simulink model "Labaa3"  (R2017b)
settings: Solver=VariableStepAuto  StartTime=0.0  StopTime=10.0  RelTol=1e-3
undefined symbols (not defined in the file): qammod
libraries: commfilt2 x2, commchan3 x1, commrflib2 x1, dspsigops x1, dspstat3 x1, commsink2 x1, commrandsrc3 x1
settings Model: Creator=Дима  LastModifiedBy=Lab
settings DataIOCC: ReturnWorkspaceOutputs=on
settings DebuggingCC: UnconnectedInputMsg=none  UnconnectedOutputMsg=none  UnconnectedLineMsg=none
settings ModelReferenceCC: EnableRefExpFcnMdlSchedulingChecks=off
settings SFSimCC: SimUseLocalCustomCode=on
settings RTWCC: Description=Generic Real-Time Target  RTWUseLocalCustomCode=on

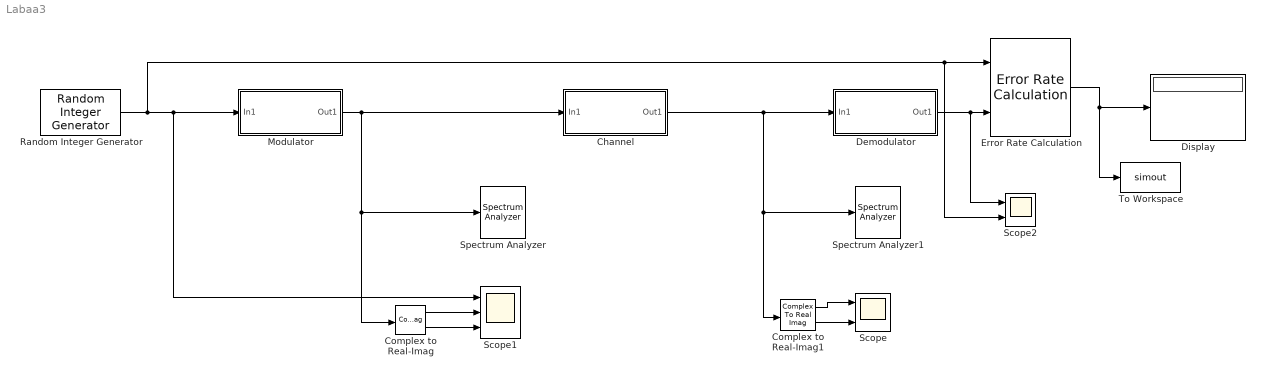
== system Labaa3 ==
  Channel : Subsystem
  Complex to Real-Imag : ComplexToRealImag
  Complex to Real-Imag1 : ComplexToRealImag
  Demodulator : Subsystem
  Display : Display
  Error Rate Calculation : commsink2/Error Rate Calculation  N=0  st_delay=0  cp_mode=Entire frame  subframe=[]  PMode=Port  WsName=ErrorVec  RsMode2=off  stop=off  numErr=100  maxBits=1e6
  Modulator : Subsystem
  Random Integer Generator : commrandsrc3/Random Integer Generator  SetSize=8  SeedSource=Auto  Seed=0  SampleTime=1/9600  SamplesPerFrame=1  OutputDataType=double  SimulateUsing=Interpreted execution
  Scope : Scope  NumInputPorts=2
  Scope1 : Scope  NumInputPorts=3
  Scope2 : Scope  NumInputPorts=2
  Spectrum Analyzer : SpectrumAnalyzer
  Spectrum Analyzer1 : SpectrumAnalyzer
  To Workspace : ToWorkspace  VariableName=simout  SaveFormat=Timeseries  SampleTime=-1
  wires:
  Complex to Real-Imag1/2 -> Scope/2
  Complex to Real-Imag1/1 -> Scope/1
  Modulator/1(Out1) -> Channel/1(In1), Complex to Real-Imag/1, Spectrum Analyzer/1
  Random Integer Generator/1 -> Scope2/2, Error Rate Calculation/1, Modulator/1(In1), Scope1/1
  Complex to Real-Imag/2 -> Scope1/3
  Complex to Real-Imag/1 -> Scope1/2
  Channel/1(Out1) -> Demodulator/1(In1), Complex to Real-Imag1/1, Spectrum Analyzer1/1
  Demodulator/1(Out1) -> Scope2/1, Error Rate Calculation/2
  Error Rate Calculation/1 -> To Workspace/1, Display/1

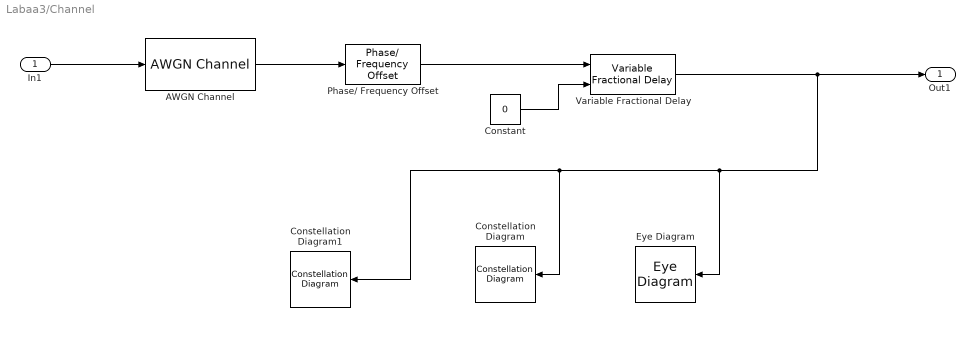
== system Labaa3/Channel ==
  In1 : Inport
  AWGN Channel : commchan3/AWGN Channel  InputProcessing=Inherited (this choice will be removed - see release notes)  seed=67  noiseMode="Signal to noise ratio  (SNR)"  EbNodB=10  EsNodB=10  SNRdB=13  bitsPerSym=1  Ps=1  Tsym=1  variance=1
  Constant : Constant  Value=0
  Constellation Diagram : ConstellationDiagram
  Constellation Diagram1 : ConstellationDiagram
  Eye Diagram : EyeDiagram
  Phase/ Frequency Offset : commrflib2/Phase// Frequency Offset  phaseOffset=0  freqPort=off  freqOffset=0
      settings: SourceProductName=Communications System Toolbox
  Variable Fractional Delay : dspsigops/Variable Fractional Delay  mode=OBSOLETE  modeActive=Linear  dmax=100  InputProcessing=Columns as channels (frame based)  L=4  FarrowL=4  R=10  alpha=1  ic=0  fallbackFIR=Clip to the minimum value necessary for centered kernel  fallbackFarrow=Clip to the minimum value necessary for centered kernel  noDFT=off  roundingMode=Zero  overflowMode=off
      settings: SourceProductName=DSP System Toolbox  SourceProductBaseCode=DS
  Out1 : Outport  VectorParamsAs1DForOutWhenUnconnected=on
  wires:
  In1/1 -> AWGN Channel/1
  AWGN Channel/1 -> Phase/ Frequency Offset/1
  Phase/ Frequency Offset/1 -> Variable Fractional Delay/1
  Constant/1 -> Variable Fractional Delay/2
  Variable Fractional Delay/1 -> Constellation Diagram/1, Constellation Diagram1/1, Eye Diagram/1, Out1/1

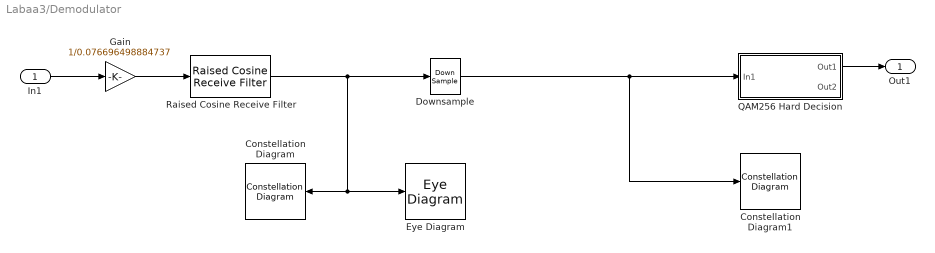
== system Labaa3/Demodulator ==
  In1 : Inport
  Constellation Diagram : ConstellationDiagram
  Constellation Diagram1 : ConstellationDiagram
  Downsample : DownSample  N=8  RateOptions=Allow multirate processing
  Eye Diagram : EyeDiagram
  Gain : Gain  Gain=1/0.076696498884737
  QAM256 Hard Decision : Subsystem
  Raised Cosine Receive Filter : commfilt2/Raised Cosine Receive Filter  filtType=Square root  R=0.8  filtSpan=10  N=8  downFactor=8  downOffset=0  filterGain=1  RateOptions=Allow multirate processing  framing=Mute  checkCoeff=off  variableName=rcRxFilt  currentFiltSpan=10  D=5  inputOffset=0  sampMode=Mute  saveAsFlag=0  rateMode=Downsampling  checkGain=Normalized  launchFVT=on  roundingMode=Floor  overflowMode=off  coeffDataTypeStr=Inherit: Same word length as input  coeffMin=[]  coeffMax=[]  coeffLastDataTypeStr=Inherit: Same word length as input  accumDataTypeStr=Inherit: Same as product output  accumLastDataTypeStr=Inherit: Same as product output  outputDataTypeStr=Inherit: Same as accumulator  outputMin=[]  outputMax=[]  outputLastDataTypeStr=Inherit: Same as accumulator
  Out1 : Outport  VectorParamsAs1DForOutWhenUnconnected=on
  wires:
  In1/1 -> Gain/1
  Gain/1 -> Raised Cosine Receive Filter/1
  Raised Cosine Receive Filter/1 -> Constellation Diagram/1, Eye Diagram/1, Downsample/1
  Downsample/1 -> Constellation Diagram1/1, QAM256 Hard Decision/1(In1)
  QAM256 Hard Decision/1(Out1) -> Out1/1

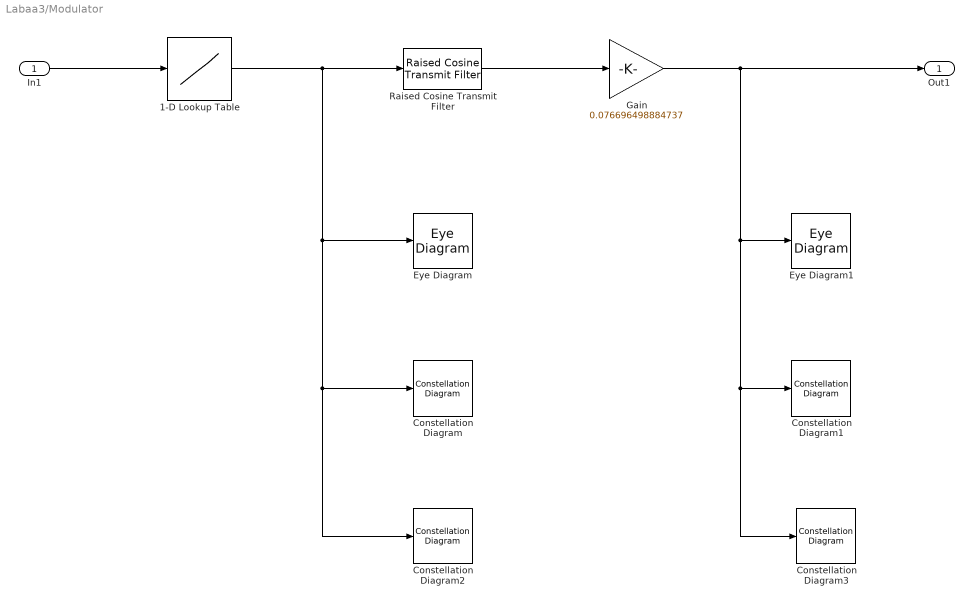
== system Labaa3/Modulator ==
  In1 : Inport
  1-D Lookup Table : Lookup_n-D  NumberOfTableDimensions=1  BreakpointsForDimension1=[0:1:255]  Table=qammod([0:1:255],256)  InternalRulePriority=Speed
  Constellation Diagram{,1..3} (4 alike) : ConstellationDiagram
  Eye Diagram : EyeDiagram
  Eye Diagram1 : EyeDiagram
  Gain : Gain  Gain=0.076696498884737
  Raised Cosine Transmit Filter : commfilt2/Raised Cosine Transmit Filter  filtType=Square root  R=0.8  filtSpan=10  N=8  filterGain=1  RateOptions=Allow multirate processing  framing=Mute  checkCoeff=off  variableName=rcTxFilt  checkGain=Normalized  sampMode=Mute  saveAsFlag=0  currentFiltSpan=10  D=(10)/2  launchFVT=on  roundingMode=Floor  overflowMode=off  coeffDataTypeStr=Inherit: Same word length as input  coeffMin=[]  coeffMax=[]  coeffLastDataTypeStr=Inherit: Same word length as input  outputDataTypeStr=Inherit: Same as accumulator  outputMin=[]  outputMax=[]  outputLastDataTypeStr=Inherit: Same as accumulator
  Out1 : Outport  VectorParamsAs1DForOutWhenUnconnected=on
  wires:
  Gain/1 -> Out1/1, Eye Diagram1/1, Constellation Diagram1/1, Constellation Diagram3/1
  In1/1 -> 1-D Lookup Table/1
  1-D Lookup Table/1 -> Raised Cosine Transmit Filter/1, Eye Diagram/1, Constellation Diagram/1, Constellation Diagram2/1
  Raised Cosine Transmit Filter/1 -> Gain/1

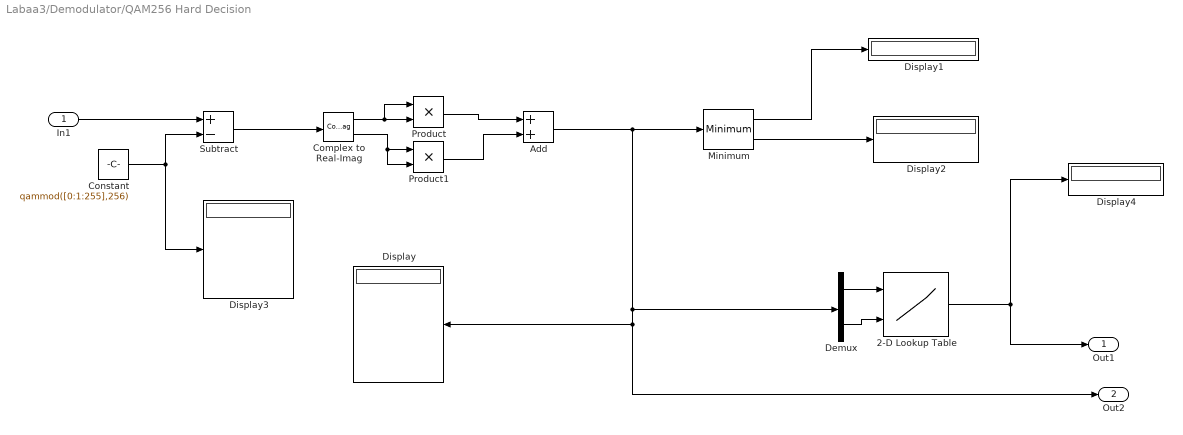
== system Labaa3/Demodulator/QAM256 Hard Decision ==
  In1 : Inport
  2-D Lookup Table : Lookup_n-D  BreakpointsForDimension1=[1:3]  BreakpointsForDimension2=[1:3]  InternalRulePriority=Speed  RndMeth=Simplest  InputSameDT=on
  Add : Sum
  Complex to Real-Imag : ComplexToRealImag
  Constant : Constant  Value=qammod([0:1:255],256)  VectorParams1D=off
  Demux : Demux  Outputs=2
  Display{,1..4} (5 alike) : Display
      Display2 settings: Format=decimal (Stored Integer)
  Minimum : dspstat3/Minimum  operation=minimum  fcn=Value and Index  indexBase=One  operateOver=Entire input  Dimension=1  InputProcessing=Columns as channels (frame based)  reset=None  roiEnable=off  roiType=Rectangles  roiPortion=Entire ROI  roiOutput=Individual statistics for each ROI  roiFlag=off  roundingMode=Floor  overflowMode=off  accumDataTypeStr=Inherit: Same as product output  accumLastDataTypeStr=Inherit: Same as product output
      settings: SourceProductName=DSP System Toolbox  SourceProductBaseCode=DS
  Product : Product
  Product1 : Product
  Subtract : Sum  Inputs=+-
  Out1 : Outport  VectorParamsAs1DForOutWhenUnconnected=on
  Out2 : Outport  Port=2  VectorParamsAs1DForOutWhenUnconnected=on
  wires:
  In1/1 -> Subtract/1
  Constant/1 -> Subtract/2, Display3/1
  Subtract/1 -> Complex to Real-Imag/1
  Product/1 -> Add/1
  Product1/1 -> Add/2
  Add/1 -> Demux/1, Out2/1, Display/1, Minimum/1
  Demux/1 -> 2-D Lookup Table/1
  Demux/2 -> 2-D Lookup Table/2
  2-D Lookup Table/1 -> Out1/1, Display4/1
  Minimum/1 -> Display1/1
  Complex to Real-Imag/1 -> Product/1, Product/2
  Complex to Real-Imag/2 -> Product1/2, Product1/1
  Minimum/2 -> Display2/1
